simulink model "SLS_Simu"  (R2021a)
settings: Solver=VariableStepAuto  StartTime=0.0  StopTime=10.0  MaxStep=1e-3  RelTol=1e-3
settings Model: Creator=Admin  LastModifiedBy=Admin
settings SolverCC: ZeroCrossControl=EnableAll

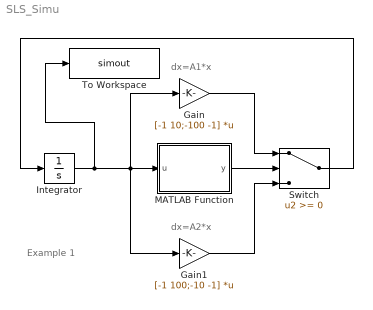
== system SLS_Simu ==
  note: Example 1
  note: dx=A1*x
  note: dx=A2*x
  Gain : Gain  Gain=[-1 10;-100 -1]  Multiplication=Matrix(K*u)
  Gain1 : Gain  Gain=[-1 100;-10 -1]  Multiplication=Matrix(K*u)
  Integrator : Integrator  InitialCondition=[10;10]
  MATLAB Function : MATLAB Function  TreatAsAtomicUnit=on
  Switch : Switch
  To Workspace : ToWorkspace  VariableName=simout  SaveFormat=Structure With Time  SampleTime=-1
  wires:
  MATLAB Function/1(y) -> Switch/2
  Switch/1 -> Integrator/1
  Integrator/1 -> To Workspace/1, Gain1/1, Gain/1, MATLAB Function/1(u)
  Gain/1 -> Switch/1
  Gain1/1 -> Switch/3

== matlab function SLS_Simu/MATLAB Function ==
  data: u input; y output
function y = fcn(u)

y = u(1)*u(2);
